simulink model "Simple_Model_v2_VISUAL"  (R2023a)
settings: Solver=VariableStepAuto  StartTime=0.0  StopTime=10.0  RelTol=1e-3
libraries: dspsigops x1
settings Model: Creator=levir  LastModifiedBy=levir

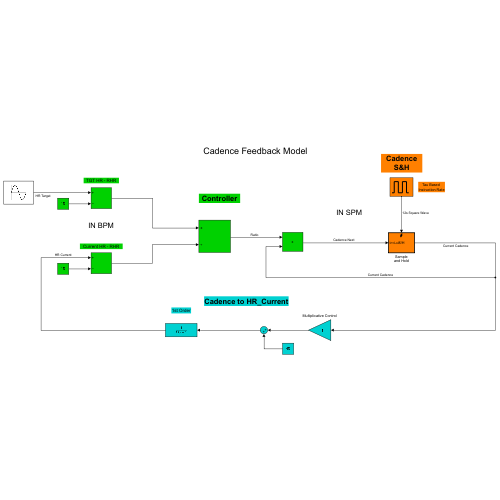
[thumbnail: Simulink's stored preview of the top-level diagram]
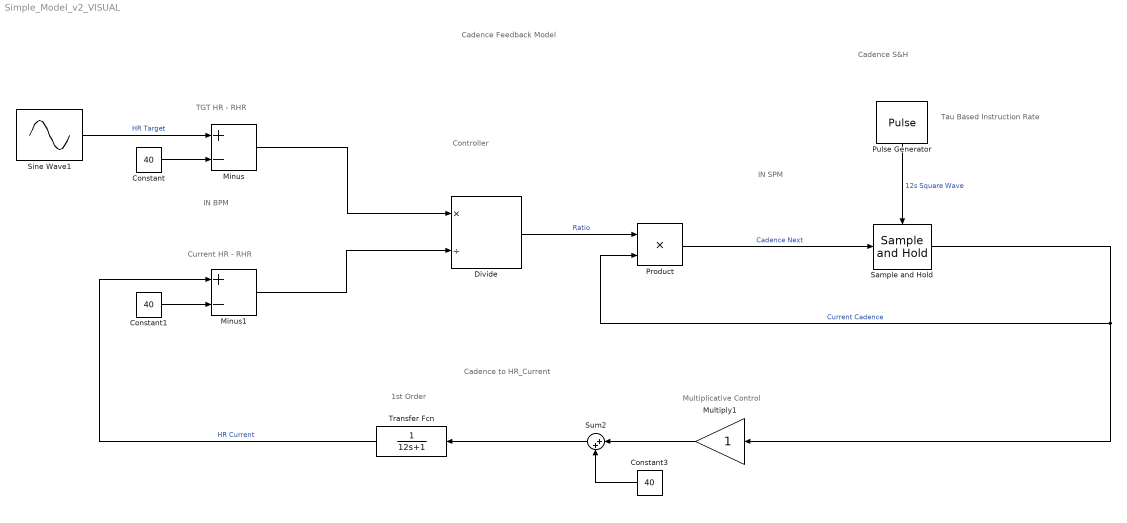
== system Simple_Model_v2_VISUAL ==
  note: Multiplicative Control
  note: Cadence to HR_Current
  note: 1st Order
  note: Tau Based
      | Instruction Rate
  note: TGT HR - RHR
  note: Cadence Feedback Model
  note: IN BPM
  note: IN SPM
  note: Current HR - RHR
  note: Controller
  note: Cadence S&H
  Constant : Constant  Value=40
  Constant1 : Constant  Value=40
  Constant3 : Constant  Value=40
  Divide : Product  Inputs=*/
  Minus : Sum  Inputs=+-
  Minus1 : Sum  Inputs=+-
  Multiply1 : Gain
  Product : Product
  Pulse Generator : DiscretePulseGenerator  PulseType=Time based  Period=12  PulseWidth=10
  Sample and Hold : dspsigops/Sample and Hold  trig=Rising edge  initCond=120  latchinput=on
  Sine Wave1 : Sin  Amplitude=20  Bias=120  Frequency=0.05  SampleTime=0
  Sum2 : Sum  Inputs=|++
  Transfer Fcn : TransferFcn  Denominator=[12 1]
  wires:
  Multiply1/1 -> Sum2/1
  Product/1 -> Sample and Hold/1  "Cadence Next"
  Sum2/1 -> Transfer Fcn/1
  Constant1/1 -> Minus1/2
  Minus/1 -> Divide/1
  Pulse Generator/1 -> Sample and Hold/Trigger  "12s Square Wave"
  Constant/1 -> Minus/2
  Constant3/1 -> Sum2/2
  Transfer Fcn/1 -> Minus1/1  "HR Current"
  Sample and Hold/1 -> Multiply1/1, Product/2  "Current Cadence"
  Minus1/1 -> Divide/2
  Sine Wave1/1 -> Minus/1  "HR Target"
  Divide/1 -> Product/1  "Ratio"
